simulink model "example19"  (R2023b)
settings: Solver=VariableStepAuto  StartTime=0.0  StopTime=10.0  RelTol=1e-3
model workspace (MAT data in the model file):
  x = 100
  y = 100
libraries: simulink x3
settings Model: Creator=ray  LastModifiedBy=ray

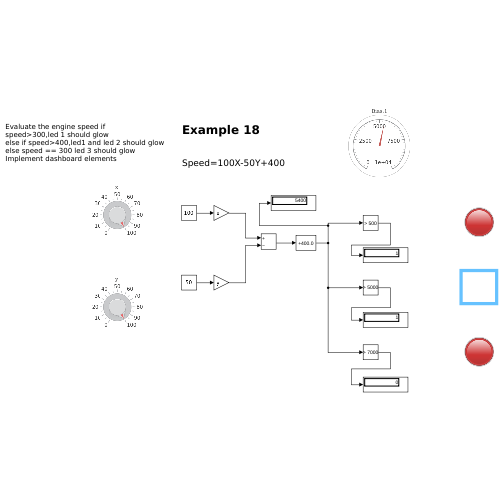
[thumbnail: Simulink's stored preview of the top-level diagram]
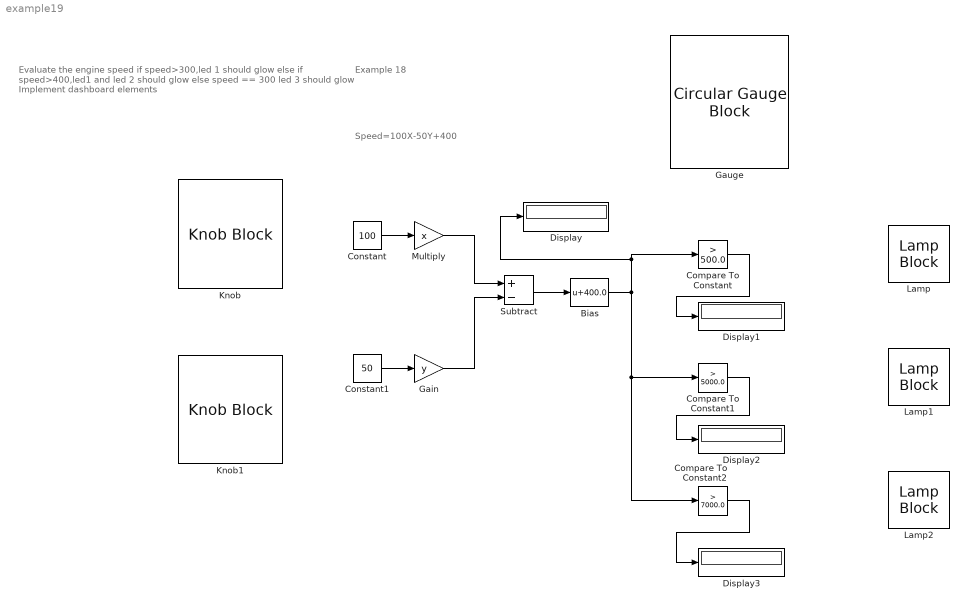
== system example19 ==
  note: Evaluate the engine speed if
      | speed>300,led 1 should glow
      | else if speed>400,led1 and led 2 should glow
      | else speed == 300 led 3 should glow
      | Implement dashboard elements
  note: Speed=100X-50Y+400
  note: Example 18
  Bias : Bias  Bias=400.0  SaturateOnIntegerOverflow=off
  Compare To Constant : simulink/Logic and Bit Operations/Compare To Constant  relop=>  const=500.0  OutDataTypeStr=boolean
  Compare To Constant1 : simulink/Logic and Bit Operations/Compare To Constant  relop=>  const=5000.0  OutDataTypeStr=boolean
  Compare To Constant2 : simulink/Logic and Bit Operations/Compare To Constant  relop=>  const=7000.0  OutDataTypeStr=boolean
  Constant : Constant  Value=100
  Constant1 : Constant  Value=50
  Display{,1..3} (4 alike) : Display
  Gain : Gain  Gain=y
  Gauge : CircularGaugeBlock  ScaleMax=10000
  Knob : KnobBlock
  Knob1 : KnobBlock
  Lamp : LampBlock  LabelPosition=Hide
  Lamp1 : LampBlock  LabelPosition=Hide
  Lamp2 : LampBlock  LabelPosition=Hide
  Multiply : Gain  Gain=x
  Subtract : Sum  Inputs=+-
  wires:
  Constant/1 -> Multiply/1
  Multiply/1 -> Subtract/1
  Constant1/1 -> Gain/1
  Gain/1 -> Subtract/2
  Subtract/1 -> Bias/1
  Bias/1 -> Display/1, Compare To Constant/1, Compare To Constant2/1, Compare To Constant1/1
  Compare To Constant/1 -> Display1/1
  Compare To Constant1/1 -> Display2/1
  Compare To Constant2/1 -> Display3/1
